simulink model "flightSimulation"  (R2025b)
settings: Solver=FixedStepAuto  StartTime=0  StopTime=10  FixedStep=Ts  RelTol=1e-3  EnableMultiTasking=on
libraries: simulink_extras x1
settings Model: Creator=The MathWorks, Inc.  LastModifiedBy=XDBDRMATION
settings SolverCC: AlgebraicLoopSolver=TrustRegion  AutoInsertRateTranBlk=on
settings DataIOCC: LimitDataPoints=on  SaveFormat=Array  SaveOutput=off  DSMLogging=off  SaveTime=off  ReturnWorkspaceOutputs=off
settings OptimizationCC: DefaultParameterBehavior=Inlined  UseDivisionForNetSlopeComputation=on  GainParamInheritBuiltInType=on  UseFloatMulNetSlope=on  OptimizeBlockIOStorage=off  ZeroExternalMemoryAtStartup=off  ZeroInternalMemoryAtStartup=off  LifeSpan=1  OptimizeDataStoreBuffers=off  BusAssignmentInplaceUpdate=off
settings DebuggingCC: AlgebraicLoopMsg=none  UnderspecifiedInitializationDetection=Classic  AllowSymbolicDim=off  PregeneratedLibrarySubsystemCodeDiagnostic=none  SFUnexpectedBacktrackingDiag=warning  SFNoUnconditionalDefaultTransitionDiag=warning  SFExecutionAtInitializationDiag=none  ArithmeticOperatorsInVariantConditions=warning
settings HardwareCC: ProdBitPerPointer=32.0  ProdBitPerSizeT=32.0  ProdBitPerPtrDiffT=32.0  ProdLargestAtomicFloat=None  ProdIntDivRoundTo=Undefined  ProdEndianess=Unspecified  ProdWordSize=32.0  ProdHWDeviceType=32-bit Generic
settings ModelReferenceCC: EnableRefExpFcnMdlSchedulingChecks=on  PropagateSignalLabelsOutOfModel=off
settings SFSimCC: SimUseLocalCustomCode=off  MATLABDynamicMemAlloc=off
settings RTWCC: GenCodeOnly=on  GenerateReport=on  RTWUseLocalCustomCode=off  BuildConfiguration=Debug  LaunchReport=on  TargetLang=C++  GPUComputeCapability=3.5
settings CodeAppCC: ForceParamTrailComments=on  MATLABSourceComments=on  EnableCustomComments=on
settings GRTTargetCC: MultiInstanceErrorCode=Warning  TargetLangStandard=C++11 (ISO)  CombineSignalStateStructs=on  CodeInterfacePackaging=C++ class  SubcomponentCodeInterfacePackaging=C++ class  SupportVariableSizeSignals=on
settings ConfigComp: CovMetricSettings=dw  CovSaveCumulativeToWorkspaceVar=on  CovSaveSingleToWorkspaceVar=on  CovExternalEMLEnable=off  CovSFcnEnable=off

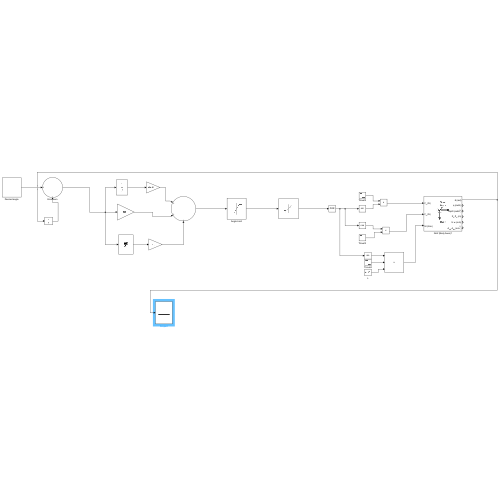
[thumbnail: Simulink's stored preview of the top-level diagram]
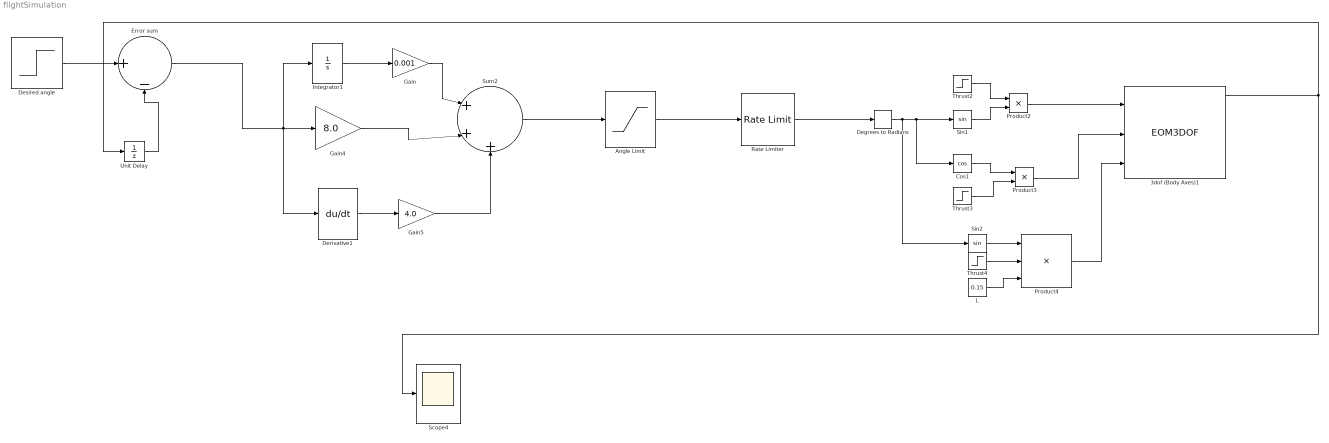
== system flightSimulation ==
  3dof (Body Axes)1 : EOM3DOF
  Angle Limit : Saturate  UpperLimit=0.2618  LowerLimit=-0.2618
  Cos1 : Trigonometry  Operator=cos
  Degrees to Radians : simulink_extras/Transformations/Degrees to Radians
  Derivative1 : Derivative
  Desired angle : Step  Before=0.3  After=0.3  SampleTime=0
  Error sum : Sum  Inputs=|+-
  Gain : Gain  Gain=0.001
  Gain4 : Gain  Gain=8.0
  Gain5 : Gain  Gain=4.0
  Integrator1 : Integrator
  L : Constant  Value=0.15
  Product2 : Product
  Product3 : Product
  Product4 : Product  Inputs=3
  Rate Limiter : RateLimiter  RisingSlewLimit=+6.54  FallingSlewLimit=-6.54  SampleTimeMode=inherited
  Scope4 : Scope
      settings: ActiveDisplayYMinimum=-3.9228397221148068  ActiveDisplayYMaximum=7.77302337706782  DataLoggingVariableName=ScopeData4
  Sin1 : Trigonometry
  Sin2 : Trigonometry
  Sum2 : Sum  Inputs=|+++
  Thrust2 : Step  Time=10  Before=100  After=0  SampleTime=0
  Thrust3 : Step  Time=10  Before=100  After=0  SampleTime=0
  Thrust4 : Step  Time=10  Before=100  After=0  SampleTime=0
  Unit Delay : UnitDelay  SampleTime=-1  HasFrameUpgradeWarning=on
  wires:
  Integrator1/1 -> Gain/1
  Derivative1/1 -> Gain5/1
  Gain/1 -> Sum2/1
  Gain4/1 -> Sum2/2
  Gain5/1 -> Sum2/3
  Error sum/1 -> Derivative1/1, Integrator1/1, Gain4/1
  Desired angle/1 -> Error sum/1
  Sum2/1 -> Angle Limit/1
  Angle Limit/1 -> Rate Limiter/1
  Rate Limiter/1 -> Degrees to Radians/1
  Degrees to Radians/1 -> Sin2/1, Cos1/1, Sin1/1
  Thrust2/1 -> Product2/1
  Sin1/1 -> Product2/2
  Cos1/1 -> Product3/1
  Thrust3/1 -> Product3/2
  Product3/1 -> 3dof (Body Axes)1/2
  Product2/1 -> 3dof (Body Axes)1/1
  Sin2/1 -> Product4/1
  Thrust4/1 -> Product4/2
  L/1 -> Product4/3
  Product4/1 -> 3dof (Body Axes)1/3
  3dof (Body Axes)1/1 -> Unit Delay/1, Scope4/1
  Unit Delay/1 -> Error sum/2
